simulink model "SistemSegOrdeCont"  (R2015b)
settings: Solver=FixedStepAuto  SolverMode=SingleTasking  StartTime=-15*(1/sqrt(40))  StopTime=40*(1/3)  FixedStep=1/10000  RelTol=1e-3
settings Model: Creator=lukit  LastModifiedBy=lukit
settings DataIOCC: LimitDataPoints=off
settings DebuggingCC: AllowSymbolicDim=on  SFUnexpectedBacktrackingDiag=error  SFNoUnconditionalDefaultTransitionDiag=error
settings ModelReferenceCC: PropagateSignalLabelsOutOfModel=on
settings SFSimCC: SimUseLocalCustomCode=on
settings RTWCC: RTWUseLocalCustomCode=on
settings GRTTargetCC: TargetLangStandard=C99 (ISO)
settings ConfigComp: CovMetricSettings=dwe  CovHtmlReporting=off  CovSaveCumulativeToWorkspaceVar=off  CovSaveSingleToWorkspaceVar=off  CovModelRefEnable=Off  CovExternalEMLEnable=on

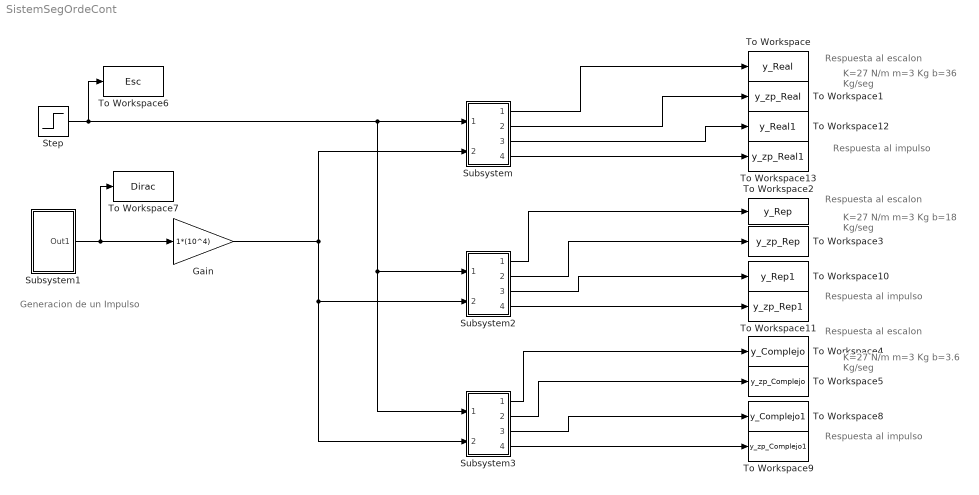
== system SistemSegOrdeCont ==
  note: Respuesta al escalon
  note: K=27 N/m
      | m=3 Kg
      | b=3.6 Kg/seg
  note: K=27 N/m
      | m=3 Kg
      | b=18 Kg/seg
  note: K=27 N/m
      | m=3 Kg
      | b=36 Kg/seg
  note: Generacion de un Impulso
  note: Respuesta al impulso
  note: Respuesta al escalon
  note: Respuesta al impulso
  note: Respuesta al escalon
  note: Respuesta al impulso
  Gain : Gain  Gain=1*(10^4)
  Step : Step  Time=0  SampleTime=0
  Subsystem : Subsystem
  Subsystem1 : Subsystem
  Subsystem2 : Subsystem
  Subsystem3 : Subsystem
  To Workspace : ToWorkspace  VariableName=y_Real  SampleTime=-1
      settings: Save2DSignal=2-D array (concatenate along first dimension)
  To Workspace1 : ToWorkspace  VariableName=y_zp_Real  SampleTime=-1
      settings: Save2DSignal=2-D array (concatenate along first dimension)
  To Workspace10 : ToWorkspace  VariableName=y_Rep1  SampleTime=-1
      settings: Save2DSignal=2-D array (concatenate along first dimension)
  To Workspace11 : ToWorkspace  VariableName=y_zp_Rep1  SampleTime=-1
      settings: Save2DSignal=2-D array (concatenate along first dimension)
  To Workspace12 : ToWorkspace  VariableName=y_Real1  SampleTime=-1
      settings: Save2DSignal=2-D array (concatenate along first dimension)
  To Workspace13 : ToWorkspace  VariableName=y_zp_Real1  SampleTime=-1
      settings: Save2DSignal=2-D array (concatenate along first dimension)
  To Workspace2 : ToWorkspace  VariableName=y_Rep  SampleTime=-1
      settings: Save2DSignal=2-D array (concatenate along first dimension)
  To Workspace3 : ToWorkspace  VariableName=y_zp_Rep  SampleTime=-1
      settings: Save2DSignal=2-D array (concatenate along first dimension)
  To Workspace4 : ToWorkspace  VariableName=y_Complejo  SampleTime=-1
      settings: Save2DSignal=2-D array (concatenate along first dimension)
  To Workspace5 : ToWorkspace  VariableName=y_zp_Complejo  SampleTime=-1
      settings: Save2DSignal=2-D array (concatenate along first dimension)
  To Workspace6 : ToWorkspace  VariableName=Esc  SampleTime=-1
      settings: Save2DSignal=2-D array (concatenate along first dimension)
  To Workspace7 : ToWorkspace  VariableName=Dirac  SampleTime=-1
      settings: Save2DSignal=2-D array (concatenate along first dimension)
  To Workspace8 : ToWorkspace  VariableName=y_Complejo1  SampleTime=-1
      settings: Save2DSignal=2-D array (concatenate along first dimension)
  To Workspace9 : ToWorkspace  VariableName=y_zp_Complejo1  SampleTime=-1
      settings: Save2DSignal=2-D array (concatenate along first dimension)
  wires:
  Subsystem/1(Out1) -> To Workspace/1
  Subsystem/2(Out2) -> To Workspace1/1
  Subsystem1/1(Out1) -> To Workspace7/1, Gain/1
  Subsystem2/1(Out1) -> To Workspace2/1
  Subsystem2/2(Out2) -> To Workspace3/1
  Gain/1 -> Subsystem/2(In2), Subsystem2/2(In2), Subsystem3/2(In2)
  Subsystem3/1(Out1) -> To Workspace4/1
  Subsystem3/2(Out2) -> To Workspace5/1
  Subsystem3/3(Out3) -> To Workspace8/1
  Subsystem3/4(Out4) -> To Workspace9/1
  Subsystem2/3(Out3) -> To Workspace10/1
  Subsystem2/4(Out4) -> To Workspace11/1
  Step/1 -> Subsystem/1(In1), Subsystem2/1(In1), Subsystem3/1(In1), To Workspace6/1
  Subsystem/3(Out3) -> To Workspace12/1
  Subsystem/4(Out4) -> To Workspace13/1

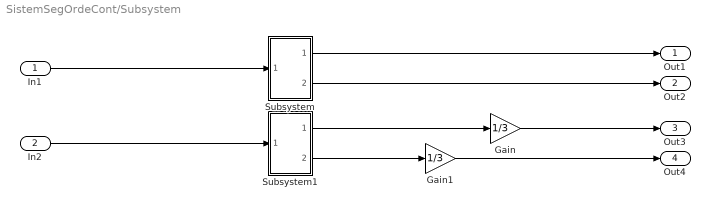
== system SistemSegOrdeCont/Subsystem ==
  In1 : Inport
  In2 : Inport  Port=2
  Gain : Gain  Gain=1/3
  Gain1 : Gain  Gain=1/3
  Subsystem : Subsystem
  Subsystem1 : Subsystem
  Out1 : Outport
  Out2 : Outport  Port=2
  Out3 : Outport  Port=3
  Out4 : Outport  Port=4
  wires:
  In1/1 -> Subsystem/1(In1)
  Subsystem/1(Out1) -> Out1/1
  Subsystem/2(Out2) -> Out2/1
  In2/1 -> Subsystem1/1(In1)
  Subsystem1/1(Out1) -> Gain/1
  Subsystem1/2(Out2) -> Gain1/1
  Gain/1 -> Out3/1
  Gain1/1 -> Out4/1

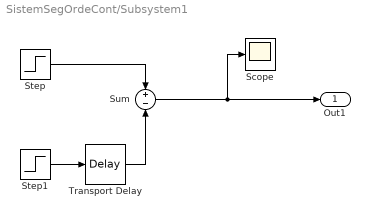
== system SistemSegOrdeCont/Subsystem1 ==
  Scope : Scope
  Step : Step  Time=0
  Step1 : Step  Time=0
  Sum : Sum  Inputs=+-
  Transport Delay : TransportDelay  DelayTime=1/10000  FixedBuffer=on
  Out1 : Outport
  wires:
  Sum/1 -> Out1/1, Scope/1
  Step1/1 -> Transport Delay/1
  Transport Delay/1 -> Sum/2
  Step/1 -> Sum/1

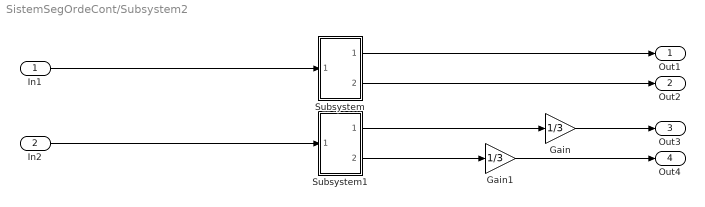
== system SistemSegOrdeCont/Subsystem2 ==
  In1 : Inport
  In2 : Inport  Port=2
  Gain : Gain  Gain=1/3
  Gain1 : Gain  Gain=1/3
  Subsystem : Subsystem
  Subsystem1 : Subsystem
  Out1 : Outport
  Out2 : Outport  Port=2
  Out3 : Outport  Port=3
  Out4 : Outport  Port=4
  wires:
  In1/1 -> Subsystem/1(In1)
  Subsystem/1(Out1) -> Out1/1
  Subsystem/2(Out2) -> Out2/1
  In2/1 -> Subsystem1/1(In1)
  Gain/1 -> Out3/1
  Subsystem1/1(Out1) -> Gain/1
  Subsystem1/2(Out2) -> Gain1/1
  Gain1/1 -> Out4/1

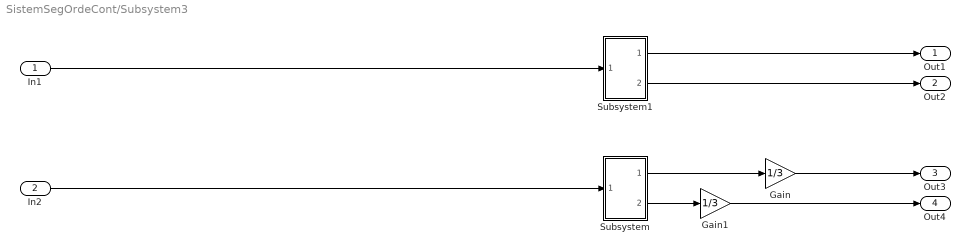
== system SistemSegOrdeCont/Subsystem3 ==
  In1 : Inport
  In2 : Inport  Port=2
  Gain : Gain  Gain=1/3
  Gain1 : Gain  Gain=1/3
  Subsystem : Subsystem
  Subsystem1 : Subsystem
  Out1 : Outport
  Out2 : Outport  Port=2
  Out3 : Outport  Port=3
  Out4 : Outport  Port=4
  wires:
  In2/1 -> Subsystem/1(In2)
  In1/1 -> Subsystem1/1(In1)
  Subsystem1/1(Out1) -> Out1/1
  Subsystem1/2(Out2) -> Out2/1
  Subsystem/1(Out3) -> Gain/1
  Gain/1 -> Out3/1
  Subsystem/2(Out4) -> Gain1/1
  Gain1/1 -> Out4/1

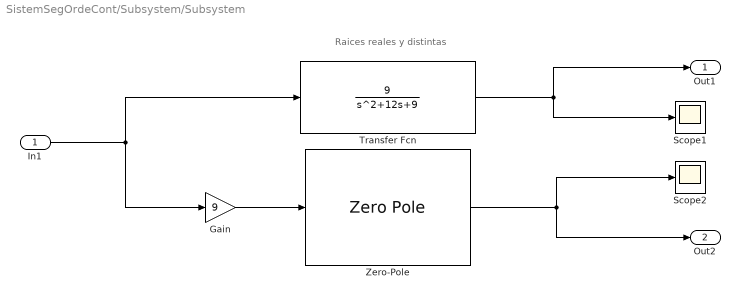
== system SistemSegOrdeCont/Subsystem/Subsystem ==
  note: Raices reales y distintas
  In1 : Inport
  Gain : Gain  Gain=9
  Scope1 : Scope
  Scope2 : Scope
  Transfer Fcn : TransferFcn  Numerator=[0,0,9]  Denominator=[1,12,9]
  Zero-Pole : ZeroPole  Zeros=[]  Poles=[-11.1962, -0.8038]
  Out1 : Outport
  Out2 : Outport  Port=2
  wires:
  In1/1 -> Gain/1, Transfer Fcn/1
  Transfer Fcn/1 -> Out1/1, Scope1/1
  Zero-Pole/1 -> Out2/1, Scope2/1
  Gain/1 -> Zero-Pole/1

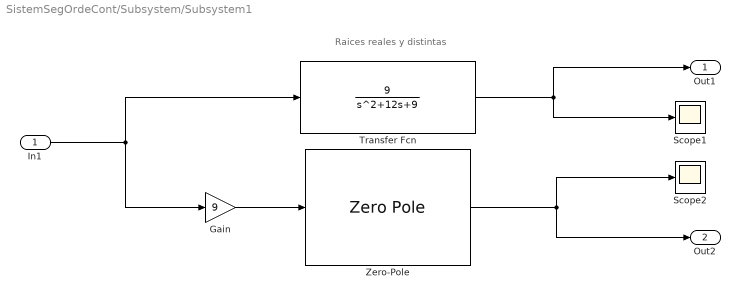
== system SistemSegOrdeCont/Subsystem/Subsystem1 ==
  note: Raices reales y distintas
  In1 : Inport
  Gain : Gain  Gain=9
  Scope1 : Scope
  Scope2 : Scope
  Transfer Fcn : TransferFcn  Numerator=[0,0,9]  Denominator=[1,12,9]
  Zero-Pole : ZeroPole  Zeros=[]  Poles=[-11.1962, -0.8038]
  Out1 : Outport
  Out2 : Outport  Port=2
  wires:
  In1/1 -> Gain/1, Transfer Fcn/1
  Transfer Fcn/1 -> Out1/1, Scope1/1
  Zero-Pole/1 -> Out2/1, Scope2/1
  Gain/1 -> Zero-Pole/1

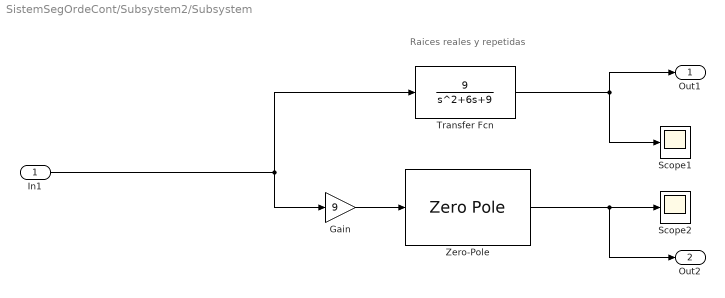
== system SistemSegOrdeCont/Subsystem2/Subsystem ==
  note: Raices reales y repetidas
  In1 : Inport
  Gain : Gain  Gain=9
  Scope1 : Scope
  Scope2 : Scope
  Transfer Fcn : TransferFcn  Numerator=[0,0,9]  Denominator=[1,6,9]
  Zero-Pole : ZeroPole  Zeros=[]  Poles=[-3, -3]
  Out1 : Outport
  Out2 : Outport  Port=2
  wires:
  Gain/1 -> Zero-Pole/1
  Zero-Pole/1 -> Out2/1, Scope2/1
  In1/1 -> Transfer Fcn/1, Gain/1
  Transfer Fcn/1 -> Out1/1, Scope1/1

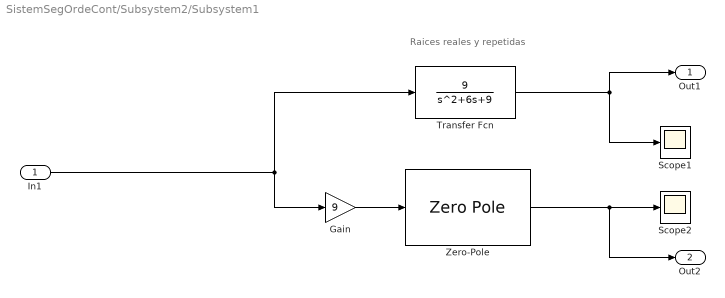
== system SistemSegOrdeCont/Subsystem2/Subsystem1 ==
  note: Raices reales y repetidas
  In1 : Inport
  Gain : Gain  Gain=9
  Scope1 : Scope
  Scope2 : Scope
  Transfer Fcn : TransferFcn  Numerator=[0,0,9]  Denominator=[1,6,9]
  Zero-Pole : ZeroPole  Zeros=[]  Poles=[-3, -3]
  Out1 : Outport
  Out2 : Outport  Port=2
  wires:
  Gain/1 -> Zero-Pole/1
  Zero-Pole/1 -> Out2/1, Scope2/1
  In1/1 -> Transfer Fcn/1, Gain/1
  Transfer Fcn/1 -> Out1/1, Scope1/1

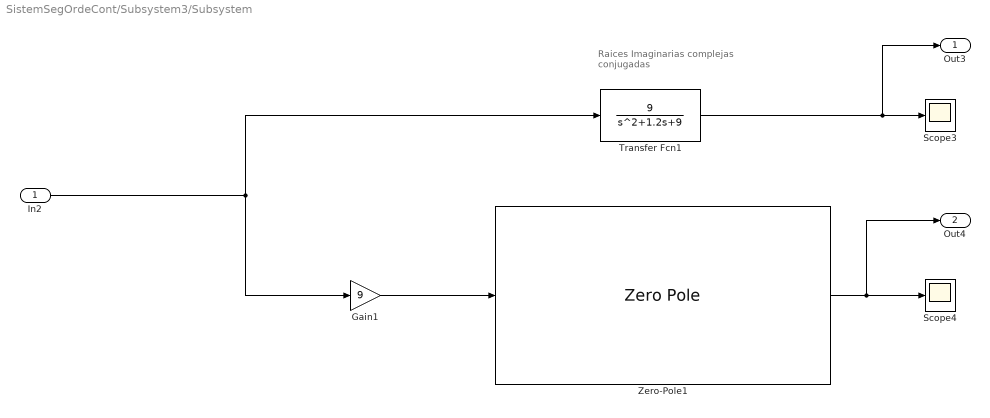
== system SistemSegOrdeCont/Subsystem3/Subsystem ==
  note: Raices Imaginarias
      |  complejas conjugadas
  In2 : Inport
  Gain1 : Gain  Gain=9
  Scope3 : Scope
  Scope4 : Scope
  Transfer Fcn1 : TransferFcn  Numerator=[0,0,9]  Denominator=[1,1.2,9]
  Zero-Pole1 : ZeroPole  Zeros=[]  Poles=[(-0.6000+2.9394i), (-0.6000-2.9394i)]
  Out3 : Outport
  Out4 : Outport  Port=2
  wires:
  Zero-Pole1/1 -> Out4/1, Scope4/1
  Transfer Fcn1/1 -> Out3/1, Scope3/1
  In2/1 -> Transfer Fcn1/1, Gain1/1
  Gain1/1 -> Zero-Pole1/1

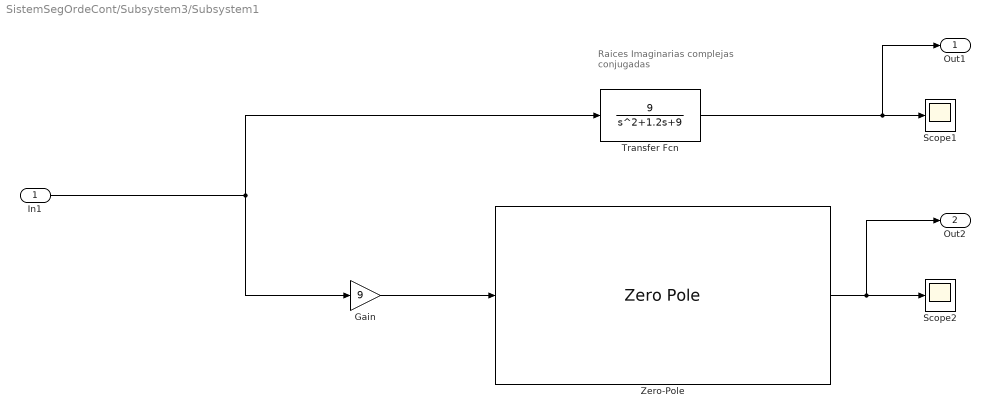
== system SistemSegOrdeCont/Subsystem3/Subsystem1 ==
  note: Raices Imaginarias
      |  complejas conjugadas
  In1 : Inport
  Gain : Gain  Gain=9
  Scope1 : Scope
  Scope2 : Scope
  Transfer Fcn : TransferFcn  Numerator=[0,0,9]  Denominator=[1,1.2,9]
  Zero-Pole : ZeroPole  Zeros=[]  Poles=[(-0.6000+2.9394i), (-0.6000-2.9394i)]
  Out1 : Outport
  Out2 : Outport  Port=2
  wires:
  Transfer Fcn/1 -> Out1/1, Scope1/1
  In1/1 -> Transfer Fcn/1, Gain/1
  Gain/1 -> Zero-Pole/1
  Zero-Pole/1 -> Out2/1, Scope2/1
